simulink model "model_one"  (R2015b)
settings: Solver=VariableStepAuto  StartTime=0.0  StopTime=10  RelTol=1e-3
libraries: simulink x1
settings Model: Creator=nlsnj  LastModifiedBy=nlsnj

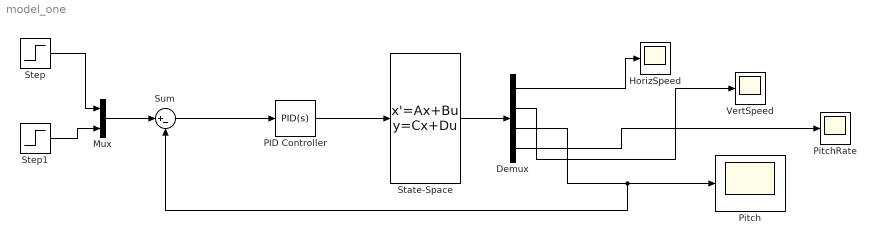
== system model_one ==
  Demux : Demux
  HorizSpeed : Scope
  Mux : Mux  Inputs=2
  PID Controller : simulink/Continuous/PID Controller  Controller=PID  TimeDomain=Continuous-time  SampleTime=-1  IntegratorMethod=Forward Euler  FilterMethod=Forward Euler  Form=Parallel  UseFilter=on  ControllerParametersSource=internal  P=1  I=1  D=0  N=100  InitialConditionSource=internal  InitialConditionForIntegrator=0  InitialConditionForFilter=0  ExternalReset=none  LimitOutput=off  UpperSaturationLimit=inf  LowerSaturationLimit=-inf  LinearizeAsGain=on  AntiWindupMode=none  Kb=1  TrackingMode=off  Kt=1  PParamMin=[]  PParamMax=[]  IParamMin=[]  IParamMax=[]  DParamMin=[]  DParamMax=[]  NParamMin=[]  NParamMax=[]  KbParamMin=[]  KbParamMax=[]  KtParamMin=[]  KtParamMax=[]  POutMin=[]  POutMax=[]  IOutMin=[]  IOutMax=[]  DOutMin=[]  DOutMax=[]  NOutMin=[]  NOutMax=[]  KbOutMin=[]  KbOutMax=[]  KtOutMin=[]  KtOutMax=[]  IntegratorOutMin=[]  IntegratorOutMax=[]  FilterOutMin=[]  FilterOutMax=[]  SumOutMin=[]  SumOutMax=[]  SumI1OutMin=[]  SumI1OutMax=[]  SumI2OutMin=[]  SumI2OutMax=[]  SumI3OutMin=[]  SumI3OutMax=[]  SumDOutMin=[]  SumDOutMax=[]  SaturationOutMin=[]  SaturationOutMax=[]  IntegratorContinuousStateAttributes=''  IntegratorStateMustResolveToSignalObject=off  IntegratorRTWStateStorageClass=Auto  FilterContinuousStateAttributes=''  FilterStateMustResolveToSignalObject=off  FilterRTWStateStorageClass=Auto  DifferentiatorICPrevScaledInput=0  DifferentiatorOutMin=[]  DifferentiatorOutMax=[]
  Pitch : Scope
  PitchRate : Scope
  State-Space : StateSpace  A="[-1.55751718e-02 -7.16617193e-04  9.11529061e-01 -9.79307808e+00; -1.00162415e-01 -3.32024131e-01  5.00648416e+00  3.59298253e-03 ; 2.25814232e-03  1.14688187e-04 -1.45542130e-01  1.22643219e-32 ; 0.00000000e+00  0.00000000e+00  1.00000000e+00  0.00000000e+00 ]"  B="[-0.55521837   9.79281659 ; -84.8645314    1.68440452 ; 0.08883462  -1.56684496 ; 0.           0. ]"  C=eye(4)  D=zeros(4,2)  X0=0  ContinuousStateAttributes='xxx'
  Step : Step  Time=0  Before=0.0  After=0.0  SampleTime=0.1
  Step1 : Step  Time=5  Before=0.0  After=0.0  SampleTime=0.1
  Sum : Sum  Inputs=|+-
  VertSpeed : Scope
  wires:
  Demux/4 -> PitchRate/1
  Demux/3 -> Sum/2, Pitch/1
  Demux/2 -> VertSpeed/1
  Demux/1 -> HorizSpeed/1
  State-Space/1 -> Demux/1
  Sum/1 -> PID Controller/1
  Step1/1 -> Mux/2
  Step/1 -> Mux/1
  PID Controller/1 -> State-Space/1
  Mux/1 -> Sum/1
